simulink model "EnableTriggred_Subsystem"  (R2024b)
settings: Solver=VariableStepAuto  StartTime=0.0  StopTime=10.0  RelTol=1e-3
settings Model: Creator=Ahmad  LastModifiedBy=Ahmad

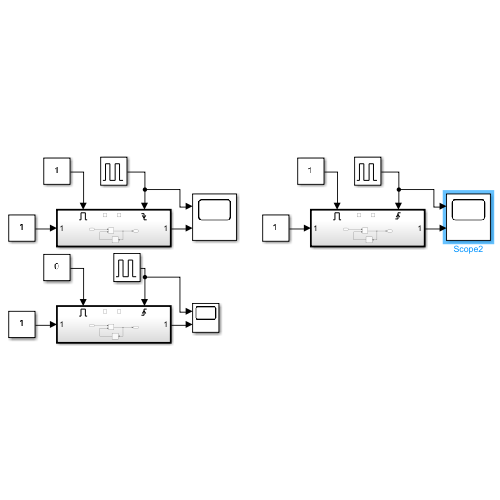
[thumbnail: Simulink's stored preview of the top-level diagram]
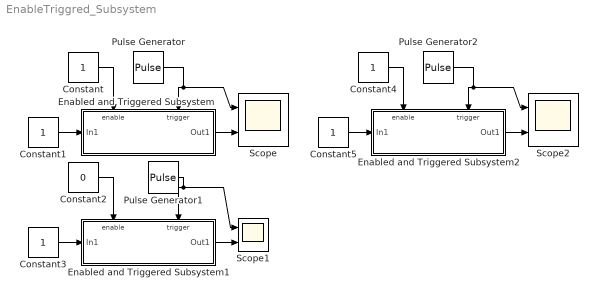
== system EnableTriggred_Subsystem ==
  Constant{,1,3..5} (5 alike) : Constant
  Constant2 : Constant  Value=0
  Enabled and Triggered Subsystem : Subsystem  TreatAsAtomicUnit=on
  Enabled and Triggered Subsystem1 : Subsystem  TreatAsAtomicUnit=on
  Enabled and Triggered Subsystem2 : Subsystem  TreatAsAtomicUnit=on
  Pulse Generator : DiscretePulseGenerator  PulseType=Time based  Period=10  PulseWidth=5
  Pulse Generator1 : DiscretePulseGenerator  PulseType=Time based  Period=10  PulseWidth=5
  Pulse Generator2 : DiscretePulseGenerator  PulseType=Time based  Period=10  PulseWidth=5  PhaseDelay=1
  Scope : Scope  NumInputPorts=2
  Scope1 : Scope  NumInputPorts=2
  Scope2 : Scope  NumInputPorts=2
  wires:
  Pulse Generator/1 -> Scope/1, Enabled and Triggered Subsystem/Trigger
  Constant1/1 -> Enabled and Triggered Subsystem/1(In1)
  Constant/1 -> Enabled and Triggered Subsystem/Enable
  Enabled and Triggered Subsystem/1(Out1) -> Scope/2
  Enabled and Triggered Subsystem1/1(Out1) -> Scope1/2
  Constant2/1 -> Enabled and Triggered Subsystem1/Enable
  Pulse Generator1/1 -> Scope1/1, Enabled and Triggered Subsystem1/Trigger
  Constant3/1 -> Enabled and Triggered Subsystem1/1(In1)
  Enabled and Triggered Subsystem2/1(Out1) -> Scope2/2
  Constant4/1 -> Enabled and Triggered Subsystem2/Enable
  Pulse Generator2/1 -> Scope2/1, Enabled and Triggered Subsystem2/Trigger
  Constant5/1 -> Enabled and Triggered Subsystem2/1(In1)

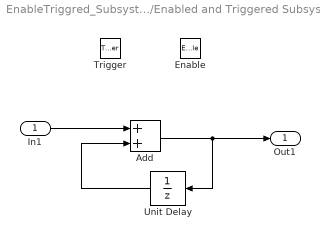
== system EnableTriggred_Subsystem/Enabled and Triggered Subsystem ==
  In1 : Inport
  Enable : EnablePort
  Trigger : TriggerPort  TriggerType=falling  VariantControl=(inherit)
  Add : Sum
  Unit Delay : UnitDelay  SampleTime=-1  HasFrameUpgradeWarning=on
  Out1 : Outport
  wires:
  In1/1 -> Add/1
  Add/1 -> Unit Delay/1, Out1/1
  Unit Delay/1 -> Add/2

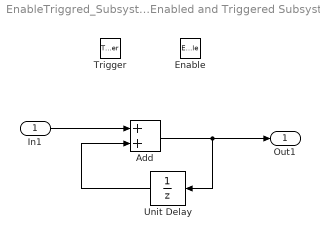
== system EnableTriggred_Subsystem/Enabled and Triggered Subsystem1 ==
  In1 : Inport
  Enable : EnablePort
  Trigger : TriggerPort  VariantControl=(inherit)
  Add : Sum
  Unit Delay : UnitDelay  SampleTime=-1  HasFrameUpgradeWarning=on
  Out1 : Outport
  wires:
  In1/1 -> Add/1
  Add/1 -> Unit Delay/1, Out1/1
  Unit Delay/1 -> Add/2

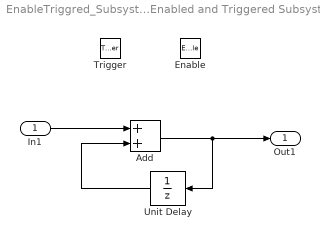
== system EnableTriggred_Subsystem/Enabled and Triggered Subsystem2 ==
  In1 : Inport
  Enable : EnablePort
  Trigger : TriggerPort  VariantControl=(inherit)
  Add : Sum
  Unit Delay : UnitDelay  SampleTime=-1  HasFrameUpgradeWarning=on
  Out1 : Outport
  wires:
  In1/1 -> Add/1
  Add/1 -> Unit Delay/1, Out1/1
  Unit Delay/1 -> Add/2
